simulink model "PID_Controller"  (R2018b)
settings: Solver=FixedStepAuto  StartTime=0.0  StopTime=10.0  FixedStep=0.01  RelTol=1e-3
settings Model: Creator=nswat  LastModifiedBy=nswat

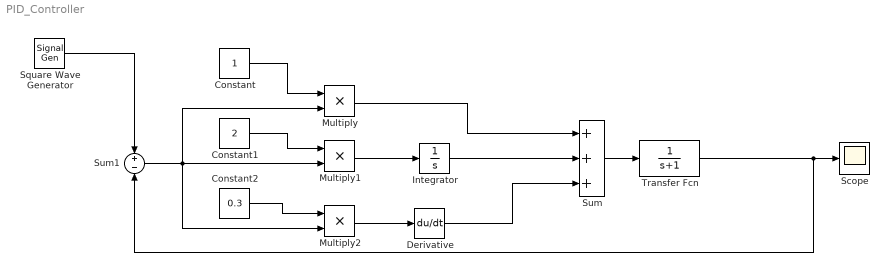
== system PID_Controller ==
  Constant : Constant
  Constant1 : Constant  Value=2
  Constant2 : Constant  Value=0.3
  Derivative : Derivative  CoefficientInTFapproximation=0
  Integrator : Integrator
  Multiply : Product
  Multiply1 : Product
  Multiply2 : Product
  Scope : Scope
  Square Wave Generator : SignalGenerator  WaveForm=square  Frequency=0.1
  Sum : Sum  Inputs=+++
  Sum1 : Sum  Inputs=+-
  Transfer Fcn : TransferFcn  Denominator=[1 1]
  wires:
  Constant/1 -> Multiply/1
  Constant1/1 -> Multiply1/1
  Constant2/1 -> Multiply2/1
  Multiply1/1 -> Integrator/1
  Multiply2/1 -> Derivative/1
  Multiply/1 -> Sum/1
  Integrator/1 -> Sum/2
  Derivative/1 -> Sum/3
  Sum/1 -> Transfer Fcn/1
  Square Wave Generator/1 -> Sum1/1
  Sum1/1 -> Multiply2/2, Multiply1/2, Multiply/2
  Transfer Fcn/1 -> Sum1/2, Scope/1
